simulink model "MRAC_function"  (R2020a)
settings: Solver=VariableStepAuto  StartTime=0.0  StopTime=100  FixedStep=0.01  RelTol=1e-3  EnableMultiTasking=on
PreLoadFcn:
  | R= 2.0; % Ohms
  | L= 0.5; % Henrys
  | Km = .015; % torque constant
  | Kb = .015; % emf constant
  | B = 0.2; % Nms
  | J= 0.02; % kg.m^2
  | Kc= 1;
  | Kf = 0.2;
  | gamma = 0.1;
values from neighbouring files (symbols this model uses):
  s = x_errdot+lambda*x_err    [ley_adapt.m]
undefined symbols (not defined in the file or in its folder): deg, InitialCondition, rad
libraries: aerolibconvert2 x8
settings Model: Creator=cpatel  LastModifiedBy=DELL
settings DataIOCC: LimitDataPoints=on  SaveFormat=Array  ReturnWorkspaceOutputs=off
settings OptimizationCC: ExpressionDepthLimit=2147483647  LifeSpan=inf
settings DebuggingCC: UnderspecifiedInitializationDetection=Classic  MergeDetectMultiDrivingBlocksExec=none  SolverPrmCheckMsg=warning  StateNameClashWarn=warning  SFUnexpectedBacktrackingDiag=warning  SFNoUnconditionalDefaultTransitionDiag=warning  SFExecutionAtInitializationDiag=none  ArithmeticOperatorsInVariantConditions=warning
settings HardwareCC: ProdBitPerPointer=32  ProdBitPerSizeT=32  ProdBitPerPtrDiffT=32  ProdLargestAtomicFloat=None  ProdIntDivRoundTo=Undefined  ProdEndianess=Unspecified  ProdWordSize=32  ProdHWDeviceType=32-bit Generic
settings ModelReferenceCC: PropagateSignalLabelsOutOfModel=off
settings SFSimCC: SimUseLocalCustomCode=off  CustomCodeUndefinedFunction=UseInterfaceOnly
settings RTWCC: RTWUseLocalCustomCode=off
settings CodeAppCC: StateflowObjectComments=on
settings GRTTargetCC: TargetLangStandard=C89/C90 (ANSI)  CombineOutputUpdateFcns=off  GRTInterface=on
settings ConfigComp: CovMetricSettings=dw  CovHtmlReporting=on  CovSaveCumulativeToWorkspaceVar=on  CovSaveSingleToWorkspaceVar=on  CovExternalEMLEnable=off

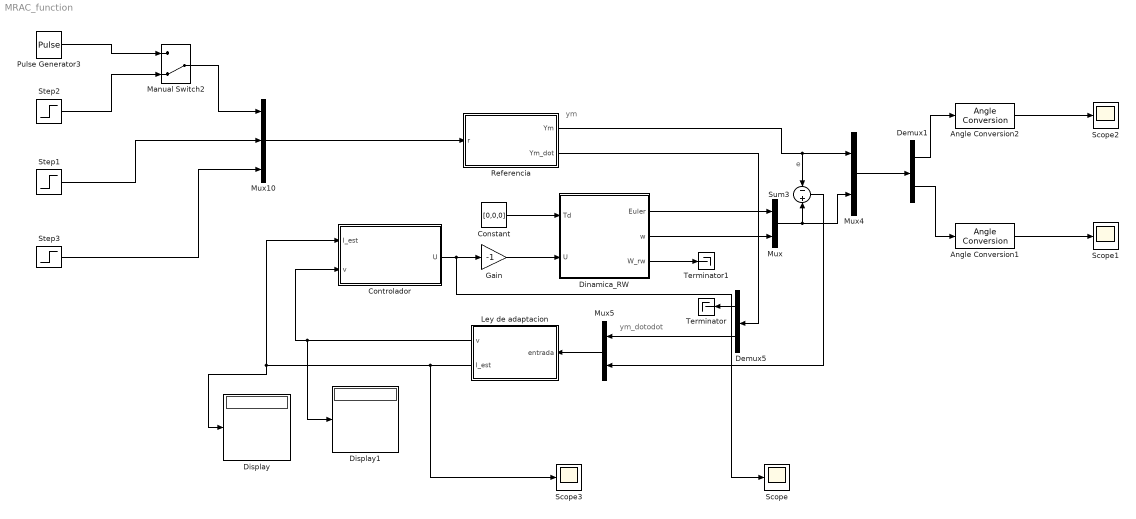
== system MRAC_function ==
  note: e
  note: ym_dotodot
  note: ym
  Angle Conversion1 : aerolibconvert2/Angle Conversion  IU=rad  OU=deg
  Angle Conversion2 : aerolibconvert2/Angle Conversion  IU=rad  OU=deg
  Constant : Constant  Value=[0,0,0]
  Controlador : Subsystem
  Demux1 : Demux  Outputs=2
  Demux5 : Demux  Outputs=2
  Dinamica_RW : Subsystem  mask{I=[8.46,8.46,8.46,1.1,1.5,1.6]*10^(-3), Ang=[0,0,0], W=[0,0,0], Wrw=[0,0,0], dimensiones=[0.015,0.025,0.043]}
      mask prompts: I "[Ix,Iy,Iz,Ixy,Ixz,Iyz] :"; Ang "[roll,pitch,yaw]:"; W "[Wx,Wy,Wz]"; Wrw "[Wrwx,Wrwy,Wrwz]"; dimensiones "[Ancho,Masa,Radio]:"
      mask TypeOptions I: I/Value
      mask TypeOptions Ang: Ang/Value
      mask TypeOptions W: W/Value
      mask TypeOptions Wrw: Wrw/Value
      mask TypeOptions dimensiones: dimentions/Value
      mask DialogControl Container3 Prompt: Tensor de Inercia
      mask DialogControl Container2 Prompt: Condiciones iniciales
      mask DialogControl Container4 Prompt: Ruedas de Reacción:
      mask DialogControl Control1 Prompt: Dimensiones:
  Display : Display
  Display1 : Display
  Gain : Gain  Gain=-1
  Ley de adaptacion : Subsystem  mask{Sigma=0.01, Lambda=6, Value=[0,0,0]}
      mask prompts: Value "I estimada:"
      mask TypeOptions Sigma: Sigma/Value
      mask TypeOptions Lambda: Lambda/Value
      mask TypeOptions Value: Iest_o/Value
  Manual Switch2 : ManualSwitch  CurrentSetting=0
  Mux : Mux  Inputs=2
  Mux10 : Mux  Inputs=3
  Mux4 : Mux  Inputs=2
  Mux5 : Mux  Inputs=2
  Pulse Generator3 : DiscretePulseGenerator  PulseType=Time based  Amplitude=10  Period=10  PulseWidth=5
  Referencia : Subsystem  mask{Eo=[0,0,0], Wo=[0,0,0]}
      mask prompts: Eo "Initial angles:"; Wo "Initial rates:"
      mask TypeOptions Eo: Initial Angles/Value
      mask TypeOptions Wo: Initial rates/Value
      mask DialogControl ParameterGroupVar Prompt: Initial Conditions
  Scope{,1..3} (4 alike) : Scope
  Step1 : Step  After=20  SampleTime=0
  Step2 : Step  After=10  SampleTime=0
  Step3 : Step  After=30  SampleTime=0
  Sum3 : Sum  Inputs=-|+
  Terminator : Terminator
  Terminator1 : Terminator
  wires:
  Constant/1 -> Dinamica_RW/1(Td)
  Mux4/1 -> Demux1/1
  Mux5/1 -> Ley de adaptacion/1(entrada)
  Ley de adaptacion/2(I_est) -> Scope3/1, Controlador/1(I_est), Display/1
  Sum3/1 -> Mux5/2
  Demux5/2 -> Mux5/1
  Referencia/1(Ym) -> Mux4/1, Sum3/1
  Ley de adaptacion/1(v) -> Display1/1, Controlador/2(v)
  Controlador/1(U) -> Scope/1, Gain/1
  Gain/1 -> Dinamica_RW/2(U)
  Step1/1 -> Mux10/2
  Step3/1 -> Mux10/3
  Manual Switch2/1 -> Mux10/1
  Step2/1 -> Manual Switch2/2
  Pulse Generator3/1 -> Manual Switch2/1
  Referencia/2(Ym_dot) -> Demux5/1
  Dinamica_RW/1(Euler) -> Mux/1
  Dinamica_RW/2("w ") -> Mux/2
  Mux/1 -> Mux4/2, Sum3/2
  Demux5/1 -> Terminator/1
  Dinamica_RW/3(W_rw) -> Terminator1/1
  Demux1/1 -> Angle Conversion2/1
  Angle Conversion2/1 -> Scope2/1
  Demux1/2 -> Angle Conversion1/1
  Angle Conversion1/1 -> Scope1/1
  Mux10/1 -> Referencia/1(r)

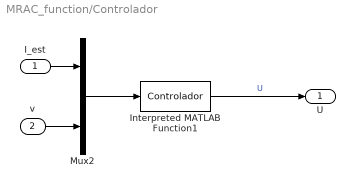
== system MRAC_function/Controlador ==
  I_est : Inport
  v : Inport  Port=2
  Interpreted MATLAB Function1 : MATLABFcn  MATLABFcn=Controlador
  Mux2 : Mux  Inputs=2
  U : Outport
  wires:
  Mux2/1 -> Interpreted MATLAB Function1/1
  v/1 -> Mux2/2
  I_est/1 -> Mux2/1
  Interpreted MATLAB Function1/1 -> U/1  "U"

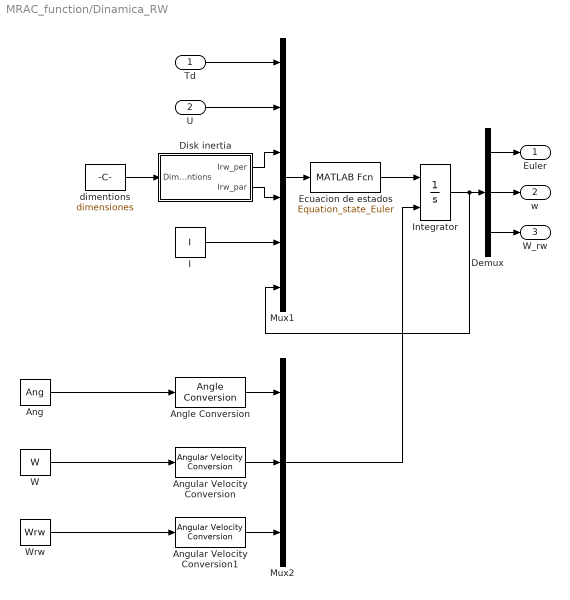
== system MRAC_function/Dinamica_RW ==
  Td : Inport
  U : Inport  Port=2
  Ang : Constant  Value=Ang
  Angle Conversion : aerolibconvert2/Angle Conversion  IU=deg  OU=rad
  Angular Velocity Conversion : aerolibconvert2/Angular Velocity Conversion  IU=deg/s  OU=rad/s
  Angular Velocity Conversion1 : aerolibconvert2/Angular Velocity Conversion  IU=deg/s  OU=rad/s
  Demux : Demux  Outputs=3
  Disk inertia : Subsystem
  Ecuacion de estados : MATLABFcn  MATLABFcn=Equation_state_Euler
  I : Constant  Value=I
  Integrator : Integrator  InitialConditionSource=external  InitialCondition=InitialCondition
  Mux1 : Mux  Inputs=6
  Mux2 : Mux  Inputs=3
  W : Constant  Value=W
  Wrw : Constant  Value=Wrw
  dimentions : Constant  Value=dimensiones
  Euler : Outport
  "w " : Outport  Port=2
  W_rw : Outport  Port=3
  wires:
  Disk inertia/2(Irw_par) -> Mux1/4
  Disk inertia/1(Irw_per) -> Mux1/3
  dimentions/1 -> Disk inertia/1(Dimentions)
  W/1 -> Angular Velocity Conversion/1
  Integrator/1 -> Demux/1, Mux1/6
  Angle Conversion/1 -> Mux2/1
  Wrw/1 -> Angular Velocity Conversion1/1
  Ang/1 -> Angle Conversion/1
  Angular Velocity Conversion/1 -> Mux2/2
  Angular Velocity Conversion1/1 -> Mux2/3
  Mux2/1 -> Integrator/2
  I/1 -> Mux1/5
  U/1 -> Mux1/2
  Mux1/1 -> Ecuacion de estados/1
  Ecuacion de estados/1 -> Integrator/1
  Td/1 -> Mux1/1
  Demux/2 -> "w "/1
  Demux/3 -> W_rw/1
  Demux/1 -> Euler/1

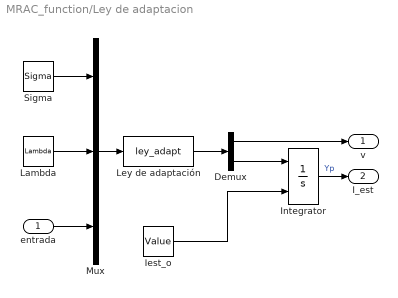
== system MRAC_function/Ley de adaptacion ==
  entrada : Inport
  Demux : Demux  Outputs=2
  Iest_o : Constant  Value=Value
  Integrator : Integrator  InitialConditionSource=external  InitialCondition=[0]
  Lambda : Constant  Value=Lambda
  Ley de adaptación : MATLABFcn  MATLABFcn=ley_adapt
  Mux : Mux  Inputs=3
  Sigma : Constant  Value=Sigma
  v : Outport
  I_est : Outport  Port=2
  wires:
  Integrator/1 -> I_est/1  "Yp"
  Ley de adaptación/1 -> Demux/1
  Demux/2 -> Integrator/1
  Demux/1 -> v/1
  Mux/1 -> Ley de adaptación/1
  entrada/1 -> Mux/3
  Sigma/1 -> Mux/1
  Lambda/1 -> Mux/2
  Iest_o/1 -> Integrator/2

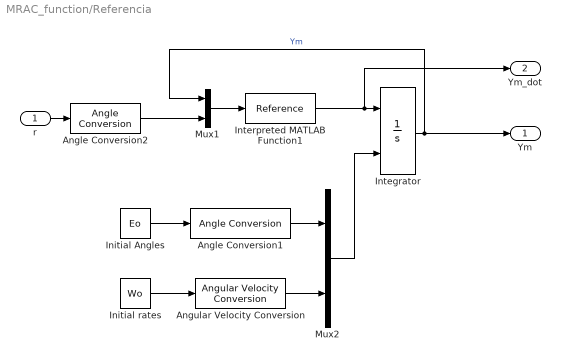
== system MRAC_function/Referencia ==
  r : Inport
  Angle Conversion1 : aerolibconvert2/Angle Conversion  IU=deg  OU=rad
  Angle Conversion2 : aerolibconvert2/Angle Conversion  IU=deg  OU=rad
  Angular Velocity Conversion : aerolibconvert2/Angular Velocity Conversion  IU=deg/s  OU=rad/s
  Initial Angles : Constant  Value=Eo
  Initial rates : Constant  Value=Wo
  Integrator : Integrator  InitialConditionSource=external  InitialCondition=[0 0]
  Interpreted MATLAB Function1 : MATLABFcn  MATLABFcn=Reference
  Mux1 : Mux  Inputs=2
  Mux2 : Mux  Inputs=2
  Ym : Outport
  Ym_dot : Outport  Port=2
  wires:
  Mux1/1 -> Interpreted MATLAB Function1/1
  Integrator/1 -> Mux1/1, Ym/1  "Ym"
  Interpreted MATLAB Function1/1 -> Ym_dot/1, Integrator/1
  Mux2/1 -> Integrator/2
  Initial Angles/1 -> Angle Conversion1/1
  Angle Conversion1/1 -> Mux2/1
  r/1 -> Angle Conversion2/1
  Angle Conversion2/1 -> Mux1/2
  Angular Velocity Conversion/1 -> Mux2/2
  Initial rates/1 -> Angular Velocity Conversion/1

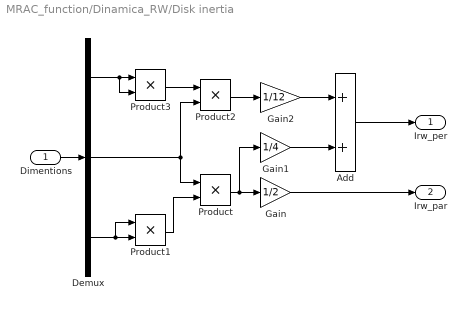
== system MRAC_function/Dinamica_RW/Disk inertia ==
  Dimentions : Inport
  Add : Sum
  Demux : Demux  Outputs=3
  Gain : Gain  Gain=1/2
  Gain1 : Gain  Gain=1/4
  Gain2 : Gain  Gain=1/12
  Product{,1..3} (4 alike) : Product
  Irw_per : Outport
  Irw_par : Outport  Port=2
  wires:
  Demux/3 -> Product1/2, Product1/1
  Dimentions/1 -> Demux/1
  Demux/2 -> Product2/2, Product/1
  Product2/1 -> Gain2/1
  Demux/1 -> Product3/1, Product3/2
  Gain/1 -> Irw_par/1
  Product1/1 -> Product/2
  Gain1/1 -> Add/2
  Add/1 -> Irw_per/1
  Product/1 -> Gain/1, Gain1/1
  Gain2/1 -> Add/1
  Product3/1 -> Product2/1
